simulink model "Trajectory"  (R2015b)
settings: Solver=VariableStepAuto  StartTime=Ts  StopTime=tsim_tra+Ts  RelTol=1e-3
values from neighbouring files (symbols this model uses):
  time_traj = 20    [Trajectory_generation.m]
  Ts = 0.01    [LQT_12states.m]    (also in Trajectory_generation.m)
  x_fin = x_traj(length(t_traj))    [Trajectory_generation.m]
  y_fin = y_traj(length(t_traj))    [Trajectory_generation.m]
undefined symbols (not defined in the file or in its folder): Discrete, Time
libraries: simulink x4, ctrlSharedLib x1, powerlib_meascontrol x1
settings Model: Creator=carlosluis  LastModifiedBy=carlosluis

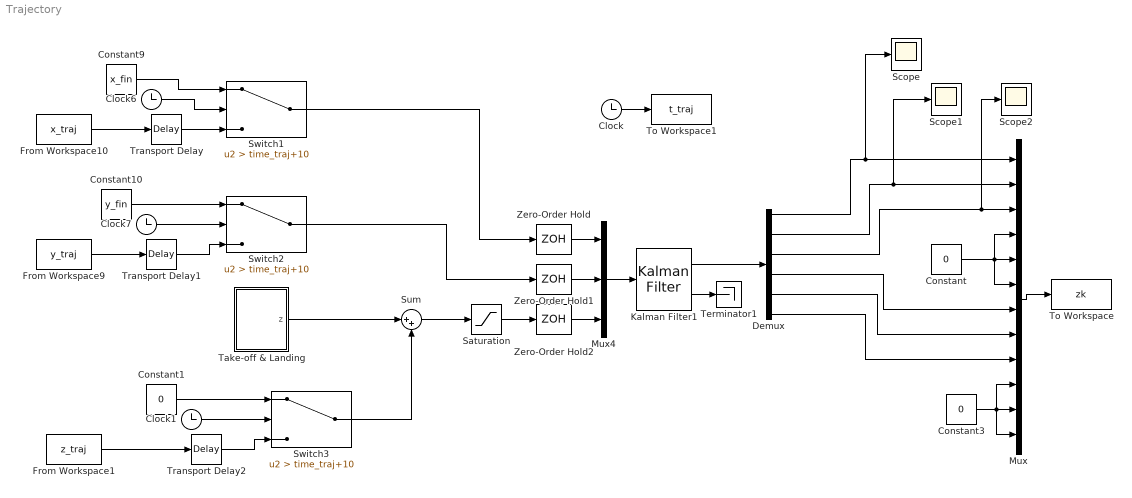
== system Trajectory ==
  Clock{,1,6..7} (4 alike) : Clock
  Constant : Constant  Value=0
  Constant1 : Constant  Value=0
  Constant10 : Constant  Value=y_fin
  Constant3 : Constant  Value=0
  Constant9 : Constant  Value=x_fin
  Demux : Demux  Outputs=6
  From Workspace1 : FromWorkspace  VariableName=z_traj  SampleTime=Ts
  From Workspace10 : FromWorkspace  VariableName=x_traj  SampleTime=Ts
  From Workspace9 : FromWorkspace  VariableName=y_traj  SampleTime=Ts
  Kalman Filter1 : ctrlSharedLib/Kalman Filter  TimeDomain=Discrete-Time  UseCurrentEstimator=on  ModelSource=Individual A, B, C, D matrices  ModelSourceVariable=ss(0.95,1,1,0,1)  A=[1 0 0 Ts 0 0; 0 1 0 0 Ts 0; 0 0 1 0 0 Ts; 0 0 0 1 0 0; 0 0 0 0 1 0; 0 0 0 0 0 1]  B=1  C=[1 0 0 0 0 0; 0 1 0 0 0 0; 0 0 1 0 0 0]  D=0  NumberOfStates=1  NumberOfInputs=1  NumberOfOutputs=1  InitialEstimateSource=Dialog  X0=0  P0=10  UseK=off  UseGH=on  NumberOfProcessNoiseInputs=1  G=[Ts/2 0 0; 0 Ts/2 0; 0 0 Ts/2; 1 0 0; 0 1 0; 0 0 1]  TimeInvariantG=on  H=0  TimeInvariantH=on  Q=diag([1 1 1])  TimeInvariantQ=on  R=0.05  TimeInvariantR=on  N=0  TimeInvariantN=on  AddInputPort=off  AddEnablePort=off  OutputEstimatedY=off  OutputP=on  Ts=Ts
  Mux : Mux  Inputs=12
  Mux4 : Mux  Inputs=3
  Saturation : Saturate  UpperLimit=2  LowerLimit=0
  Scope : Scope
  Scope1 : Scope
  Scope2 : Scope
  Sum : Sum  Inputs=|++
  Switch1 : Switch  Criteria=u2 > Threshold  Threshold=time_traj+10
  Switch2 : Switch  Criteria=u2 > Threshold  Threshold=time_traj+10
  Switch3 : Switch  Criteria=u2 > Threshold  Threshold=time_traj+10
  Take-off & Landing : Subsystem
  Terminator1 : Terminator
  To Workspace : ToWorkspace  VariableName=zk  SampleTime=Ts
  To Workspace1 : ToWorkspace  VariableName=t_traj  SampleTime=Ts
  Transport Delay : TransportDelay  DelayTime=10
  Transport Delay1 : TransportDelay  DelayTime=10
  Transport Delay2 : TransportDelay  DelayTime=10
  Zero-Order Hold : ZeroOrderHold  SampleTime=Ts
  Zero-Order Hold1 : ZeroOrderHold  SampleTime=Ts
  Zero-Order Hold2 : ZeroOrderHold  SampleTime=Ts
  wires:
  Mux/1 -> To Workspace/1
  Clock/1 -> To Workspace1/1
  Kalman Filter1/1 -> Demux/1
  Mux4/1 -> Kalman Filter1/1
  Kalman Filter1/2 -> Terminator1/1
  Zero-Order Hold/1 -> Mux4/1
  Zero-Order Hold1/1 -> Mux4/2
  Zero-Order Hold2/1 -> Mux4/3
  Constant9/1 -> Switch1/1
  Clock6/1 -> Switch1/2
  From Workspace10/1 -> Transport Delay/1
  Transport Delay/1 -> Switch1/3
  Constant10/1 -> Switch2/1
  Clock7/1 -> Switch2/2
  From Workspace9/1 -> Transport Delay1/1
  Transport Delay1/1 -> Switch2/3
  Constant1/1 -> Switch3/1
  Clock1/1 -> Switch3/2
  From Workspace1/1 -> Transport Delay2/1
  Transport Delay2/1 -> Switch3/3
  Sum/1 -> Saturation/1
  Saturation/1 -> Zero-Order Hold2/1
  Constant/1 -> Mux/5, Mux/4, Mux/6
  Take-off & Landing/1(z) -> Sum/1
  Demux/3 -> Scope2/1, Mux/3
  Demux/4 -> Mux/7
  Demux/5 -> Mux/8
  Demux/6 -> Mux/9
  Constant3/1 -> Mux/12, Mux/11, Mux/10
  Switch2/1 -> Zero-Order Hold1/1
  Switch1/1 -> Zero-Order Hold/1
  Demux/1 -> Scope/1, Mux/1
  Demux/2 -> Scope1/1, Mux/2
  Switch3/1 -> Sum/2

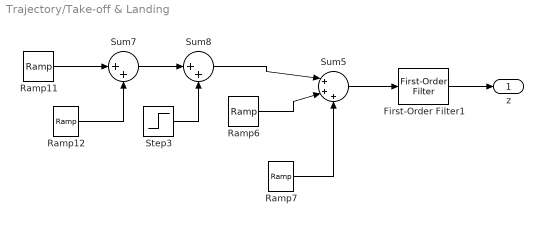
== system Trajectory/Take-off & Landing ==
  First-Order Filter1 : powerlib_meascontrol/Filters/First-Order Filter  FilterType=Lowpass  Tc=0.5  Ts=0  Initialize=on  Vac_Init=[0, 0, 60]  Vdc_Init=0  PlotResponse=off  FreqRange="[0,  200,  1]"
  Ramp11 : simulink/Sources/Ramp  slope=1/4  start=1  X0=0
  Ramp12 : simulink/Sources/Ramp  slope=-1/4  start=4  X0=0
  Ramp6 : simulink/Sources/Ramp  slope=-1/4  start=35  X0=0
  Ramp7 : simulink/Sources/Ramp  slope=1/4  start=39  X0=0
  Step3 : Step  Time=0  After=0.25  SampleTime=0
  Sum5 : Sum  Inputs=|+++
  Sum7 : Sum  Inputs=|++
  Sum8 : Sum  Inputs=|++
  z : Outport
  wires:
  Ramp6/1 -> Sum5/2
  Sum5/1 -> First-Order Filter1/1
  Ramp7/1 -> Sum5/3
  First-Order Filter1/1 -> z/1
  Ramp11/1 -> Sum7/1
  Ramp12/1 -> Sum7/2
  Sum7/1 -> Sum8/1
  Step3/1 -> Sum8/2
  Sum8/1 -> Sum5/1
